simulink model "ADAS_Brake_2_sensors_TS9"  (Simulink 7.6)
settings: Solver=ode45  SolverMode=SingleTasking  StartTime=0  StopTime=8  FixedStep=0.002  RelTol=1e-3  AbsTol=1e-6
InitFcn:
  | R2D = 180/pi;
libraries: Solver_SF x1
settings Model: Creator=pmather  LastModifiedBy=mkhan  ExtModeTrigMode=oneshot  ExtModeArmWhenConnect=off
settings DataIOCC: LimitDataPoints=off  SignalLoggingName=sigsOut
settings OptimizationCC: BlockReduction=off  BooleanDataType=off  ExpressionDepthLimit=128  InitFltsAndDblsToZero=on
settings DebuggingCC: SaveWithParameterizedLinksMsg=none  SignalResolutionControl=TryResolveAllWithWarning  SolverPrmCheckMsg=none  MultiTaskDSMMsg=warning  MultiTaskCondExecSysMsg=none  StateNameClashWarn=none  StrictBusMsg=None
settings HardwareCC: TargetUnknown=on
settings RTWCC: TemplateMakefile=grt_vc.tmf  IncludeERTFirstTime=on
settings CodeAppCC: CustomSymbolStrType=$N$R$M_T
settings GRTTargetCC: TargetFcnLib=ansi_tfl_tmw.mat

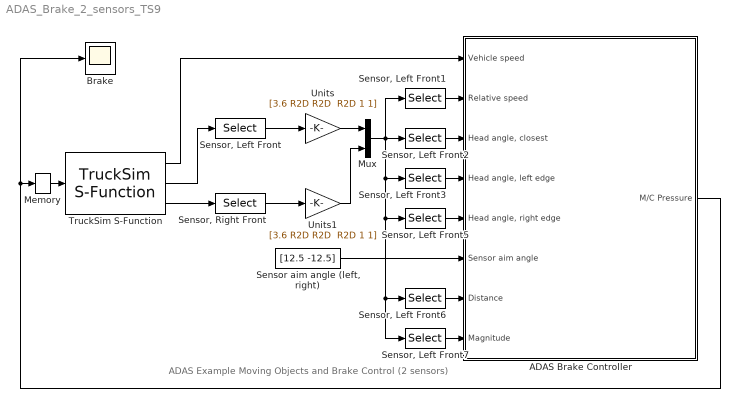
== system ADAS_Brake_2_sensors_TS9 ==
  note: ADAS Example
      | Moving Objects and Brake Control (2 sensors)
  ADAS Brake Controller : Subsystem
  Brake : Scope
      settings: TimeRange=8  YMin=0  YMax=15
  Memory : Memory
  Mux : Mux  Inputs=2
  "Sensor aim angle (left, right)" : Constant  Value=[12.5 -12.5]
  "Sensor, Left Front" : Selector  IndexOptions=Index vector (dialog)  Indices=[3 6 7 8 2 4]  OutputSizes=1
  "Sensor, Left Front1" : Selector  IndexOptions=Index vector (dialog)  Indices=[1 7]  OutputSizes=1
  "Sensor, Left Front2" : Selector  IndexOptions=Index vector (dialog)  Indices=[2 8]  OutputSizes=1
  "Sensor, Left Front3" : Selector  IndexOptions=Index vector (dialog)  Indices=[3 9]  OutputSizes=1
  "Sensor, Left Front5" : Selector  IndexOptions=Index vector (dialog)  Indices=[4 10]  OutputSizes=1
  "Sensor, Left Front6" : Selector  IndexOptions=Index vector (dialog)  Indices=[5 11]  OutputSizes=1
  "Sensor, Left Front7" : Selector  IndexOptions=Index vector (dialog)  Indices=[6 12]  OutputSizes=1
  "Sensor, Right Front" : Selector  IndexOptions=Index vector (dialog)  Indices=[3 6 7 8 2 4]  OutputSizes=1
  TruckSim S-Function : Solver_SF/TruckSim S-Function  Priority=1  SIMFILE=simfile.sim
  Units : Gain  Gain="[3.6 R2D R2D  R2D 1 1]"  SaturateOnIntegerOverflow=on  OutDataTypeStr=Inherit: Same as input  ParamDataTypeStr=Inherit: Same as input
  Units1 : Gain  Gain="[3.6 R2D R2D  R2D 1 1]"  SaturateOnIntegerOverflow=on  OutDataTypeStr=Inherit: Same as input  ParamDataTypeStr=Inherit: Same as input
  wires:
  ADAS Brake Controller/1(M/C Pressure) -> Brake/1, Memory/1
  TruckSim S-Function/1 -> ADAS Brake Controller/1(Vehicle speed)
  "Sensor, Left Front"/1 -> Units/1
  "Sensor, Right Front"/1 -> Units1/1
  Memory/1 -> TruckSim S-Function/1
  Units/1 -> Mux/1
  Units1/1 -> Mux/2
  Mux/1 -> "Sensor, Left Front1"/1, "Sensor, Left Front2"/1, "Sensor, Left Front3"/1, "Sensor, Left Front7"/1, "Sensor, Left Front6"/1, "Sensor, Left Front5"/1
  "Sensor, Left Front1"/1 -> ADAS Brake Controller/2(Relative speed)
  "Sensor, Left Front2"/1 -> ADAS Brake Controller/3("Head angle, closest")
  "Sensor, Left Front3"/1 -> ADAS Brake Controller/4("Head angle, left edge ")
  "Sensor, Left Front6"/1 -> ADAS Brake Controller/7(Distance)
  "Sensor, Left Front7"/1 -> ADAS Brake Controller/8(Magnitude)
  "Sensor, Left Front5"/1 -> ADAS Brake Controller/5("Head angle, right edge")
  "Sensor aim angle (left, right)"/1 -> ADAS Brake Controller/6(Sensor aim angle)
  TruckSim S-Function/2 -> "Sensor, Left Front"/1
  TruckSim S-Function/3 -> "Sensor, Right Front"/1

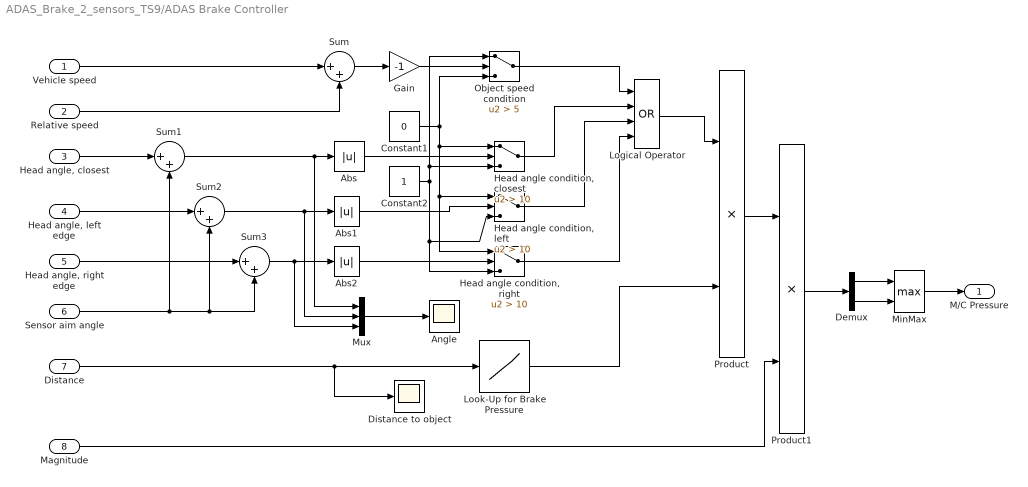
== system ADAS_Brake_2_sensors_TS9/ADAS Brake Controller ==
  Vehicle speed : Inport
  Relative speed : Inport  Port=2
  "Head angle, closest" : Inport  Port=3
  "Head angle, left edge " : Inport  Port=4
  "Head angle, right edge" : Inport  Port=5
  Sensor aim angle : Inport  Port=6
  Distance : Inport  Port=7
  Magnitude : Inport  Port=8
  Abs : Abs  SaturateOnIntegerOverflow=on
  Abs1 : Abs  SaturateOnIntegerOverflow=on
  Abs2 : Abs  SaturateOnIntegerOverflow=on
  Angle : Scope
      settings: TimeRange=8  YMin=0  YMax=25  SaveName=ScopeData3
  Constant1 : Constant  Value=0
  Constant2 : Constant
  Demux : Demux  Outputs=2
  Distance to object : Scope
      settings: TimeRange=8  YMin=0  YMax=150  SaveName=ScopeData4
  Gain : Gain  Gain=-1  SaturateOnIntegerOverflow=on  OutDataTypeStr=Inherit: Same as input  ParamDataTypeStr=Inherit: Same as input
  "Head angle condition, closest" : Switch  Criteria=u2 > Threshold  Threshold=10  SaturateOnIntegerOverflow=on
  "Head angle condition, left" : Switch  Criteria=u2 > Threshold  Threshold=10  SaturateOnIntegerOverflow=on
  "Head angle condition, right" : Switch  Criteria=u2 > Threshold  Threshold=10  SaturateOnIntegerOverflow=on
  Logical Operator : Logic  Operator=OR  Inputs=4  AllPortsSameDT=off
  Look-Up for Brake Pressure : Lookup  InputValues=[0,20,30,40,60,80,100,120]  Table=[15,15,10,10,0,0,0,0]  SaturateOnIntegerOverflow=on
  MinMax : MinMax  Function=max  Inputs=2  SaturateOnIntegerOverflow=on  InputSameDT=on
  Mux : Mux  Inputs=3
  Object speed condition : Switch  Criteria=u2 > Threshold  Threshold=5  SaturateOnIntegerOverflow=on
  Product : Product  SaturateOnIntegerOverflow=on  OutDataTypeStr=Inherit: Same as first input
  Product1 : Product  SaturateOnIntegerOverflow=on  OutDataTypeStr=Inherit: Same as first input
  Sum{,1..3} (4 alike) : Sum  Inputs=|++  SaturateOnIntegerOverflow=on
  M/C Pressure : Outport
  wires:
  Abs/1 -> "Head angle condition, closest"/2
  Constant1/1 -> Object speed condition/3, "Head angle condition, closest"/1, "Head angle condition, left"/1, "Head angle condition, right"/1
  Constant2/1 -> "Head angle condition, closest"/3, Object speed condition/1, "Head angle condition, left"/3, "Head angle condition, right"/3
  Sum/1 -> Gain/1
  Gain/1 -> Object speed condition/2
  Object speed condition/1 -> Logical Operator/1
  "Head angle condition, closest"/1 -> Logical Operator/2
  Logical Operator/1 -> Product/1
  Look-Up for Brake Pressure/1 -> Product/2
  Product/1 -> Product1/1
  Vehicle speed/1 -> Sum/1
  Relative speed/1 -> Sum/2
  Distance/1 -> Look-Up for Brake Pressure/1, Distance to object/1
  "Head angle condition, left"/1 -> Logical Operator/3
  Magnitude/1 -> Product1/2
  Mux/1 -> Angle/1
  Abs1/1 -> "Head angle condition, left"/2
  Abs2/1 -> "Head angle condition, right"/2
  "Head angle condition, right"/1 -> Logical Operator/4
  Product1/1 -> Demux/1
  Demux/1 -> MinMax/1
  Demux/2 -> MinMax/2
  MinMax/1 -> M/C Pressure/1
  "Head angle, closest"/1 -> Sum1/1
  Sum1/1 -> Abs/1, Mux/1
  Sensor aim angle/1 -> Sum1/2, Sum2/2, Sum3/2
  "Head angle, left edge "/1 -> Sum2/1
  Sum2/1 -> Abs1/1, Mux/2
  "Head angle, right edge"/1 -> Sum3/1
  Sum3/1 -> Abs2/1, Mux/3
